simulink model "Boom_Controller"  (R2020a)
settings: Solver=VariableStepAuto  StartTime=0.0  StopTime=10  RelTol=1e-3
values from neighbouring files (symbols this model uses):
  Bm = 4    [Boom_Control.m]
  Jm = 0.2    [Boom_Control.m]
  Kd = 1.5    [Boom_Control.m]
  Ke = 1.2    [Boom_Control.m]
  KI = 10    [Boom_Control.m]
  Kp = 105    [Boom_Control.m]
  Kt = 1.5    [Boom_Control.m]
  La = 0.001    [Boom_Control.m]
  r = 0.1    [Boom_Control.m]
  Ra = 0.3    [Boom_Control.m]
settings Model: Creator=alan  LastModifiedBy=alan

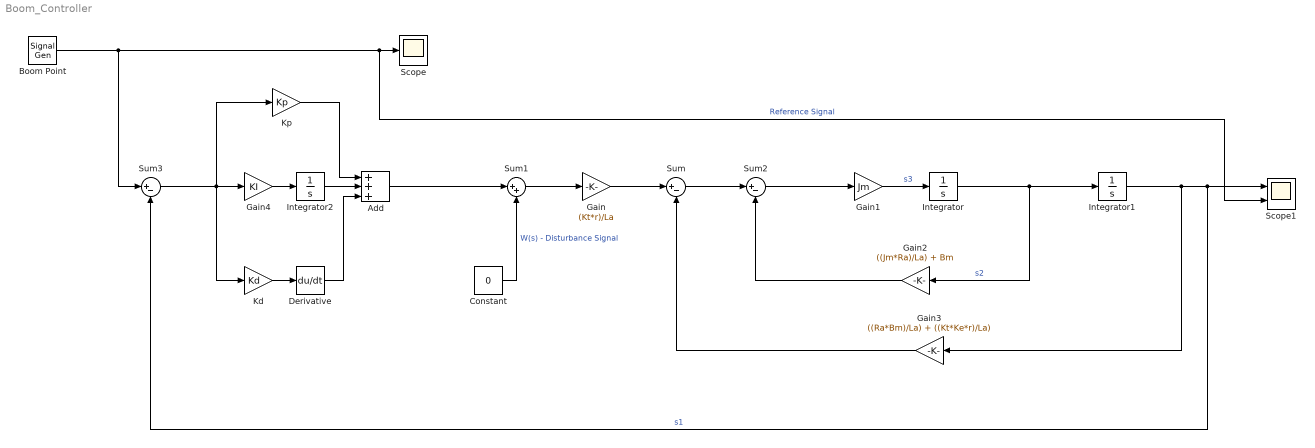
== system Boom_Controller ==
  Add : Sum  Inputs=+++
  Boom Point : SignalGenerator  Amplitude=0.3464  Frequency=2  Units=rad/sec
  Constant : Constant  Value=0
  Derivative : Derivative
  Gain : Gain  Gain=(Kt*r)/La
  Gain1 : Gain  Gain=Jm
  Gain2 : Gain  Gain=((Jm*Ra)/La) + Bm
  Gain3 : Gain  Gain=((Ra*Bm)/La) + ((Kt*Ke*r)/La)
  Gain4 : Gain  Gain=KI
  Integrator : Integrator
  Integrator1 : Integrator
  Integrator2 : Integrator
  Kd : Gain  Gain=Kd
  Kp : Gain  Gain=Kp
  Scope : Scope
  Scope1 : Scope  NumInputPorts=2
  Sum : Sum  Inputs=|+-
  Sum1 : Sum  Inputs=|++
  Sum2 : Sum  Inputs=|+-
  Sum3 : Sum  Inputs=|+-
  wires:
  Boom Point/1 -> Scope1/2, Scope/1, Sum3/1  "Reference Signal"
  Gain/1 -> Sum/1
  Gain1/1 -> Integrator/1  "s3"
  Integrator/1 -> Gain2/1, Integrator1/1  "s2"
  Sum/1 -> Sum2/1
  Sum2/1 -> Gain1/1
  Gain2/1 -> Sum2/2
  Integrator1/1 -> Gain3/1, Sum3/2, Scope1/1  "s1"
  Gain3/1 -> Sum/2
  Sum1/1 -> Gain/1
  Constant/1 -> Sum1/2  "W(s) - Disturbance Signal"
  Sum3/1 -> Gain4/1, Kd/1, Kp/1
  Kd/1 -> Derivative/1
  Kp/1 -> Add/1
  Add/1 -> Sum1/1
  Derivative/1 -> Add/3
  Gain4/1 -> Integrator2/1
  Integrator2/1 -> Add/2
